simulink library "SunEphemeris_MathWorks"  (R2014b)
settings: Solver=ode45  StartTime=0.0  StopTime=10.0  RelTol=1e-3
undefined symbols (not defined in the file or in its folder): ConfParam
settings Model: Creator=Hp  LastModifiedBy=Hp

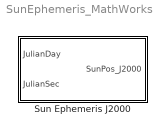
== system SunEphemeris_MathWorks ==
  Sun Ephemeris J2000 : Subsystem

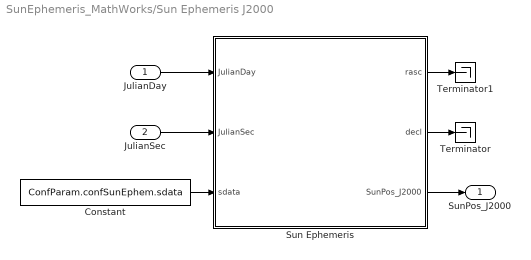
== system SunEphemeris_MathWorks/Sun Ephemeris J2000 ==
  JulianDay : Inport
  JulianSec : Inport  Port=2
  Constant : Constant  Value=ConfParam.confSunEphem.sdata
  Sun Ephemeris : MATLAB Function  TreatAsAtomicUnit=on
  Terminator : Terminator
  Terminator1 : Terminator
  SunPos_J2000 : Outport
  wires:
  Sun Ephemeris/2(decl) -> Terminator/1
  Sun Ephemeris/3(SunPos_J2000) -> SunPos_J2000/1
  JulianDay/1 -> Sun Ephemeris/1(JulianDay)
  Sun Ephemeris/1(rasc) -> Terminator1/1
  Constant/1 -> Sun Ephemeris/3(sdata)
  JulianSec/1 -> Sun Ephemeris/2(JulianSec)

== matlab function SunEphemeris_MathWorks/Sun Ephemeris J2000/Sun Ephemeris ==
  data: JulianDay input; rasc output; JulianSec input; sdata input; decl output; SunPos_J2000 output
function [rasc, decl, SunPos_J2000] = SunEphem (JulianDay, JulianSec, sdata)

% precision ephemeris of the Sun

% input
    
%  jdate = julian ephemeris date

% output

%  rasc = right ascension of the Sun (radians)
%         (0 <= rasc <= 2 pi)
%  decl = declination of the Sun (radians)
%         (-pi/2 <= decl <= pi/2)
%  rsun = eci position vector of the Sun (meters)

% note

%  coordinates are inertial, geocentric,
%  equatorial and true-of-date

% Orbital Mechanics with Matlab

%%%%%%%%%%%%%%%%%%%%%%%%%%%%%%%

sl=zeros(50,1);
sr=zeros(50,1);
sa=zeros(50,1);
sb=zeros(50,1);

% extract data and load arrays

sl(1:1:50) = sdata(1:4:200);
sr(1:1:50) = sdata(2:4:200);
sa(1:1:50) = sdata(3:4:200);
sb(1:1:50) = sdata(4:4:200);

% fundamental time argument
jdate=JulianDay+JulianSec/86400+2.4515445e6;
          
u = (jdate - 2451545) / 3652500;

% compute nutation in longitude

a1 = 2.18 + u * (-3375.7 + u * 0.36);
a2 = 3.51 + u * (125666.39 + u * 0.1);
   
psi = 0.0000001 * (-834 * sin(a1) - 64 * sin(a2));

% compute nutation in obliquity

deps = 0.0000001 * u * (-226938 + u * (-75 + u * (96926 + ...
       u * (-2491 - u * 12104))));

meps = 0.0000001 * (4090928 + 446 * cos(a1) + 28 * cos(a2));
   
eps = meps + deps;
   
seps = sin(eps);
ceps = cos(eps);

dl = 0;
dr = 0;

for i = 1:1:50
    
    w = sa(i) + sb(i) * u;
    
    dl = dl + sl(i) * sin(w);
    
    if (sr(i) ~= 0)
        
       dr = dr + sr(i) * cos(w);
       
    end 
    
end

dl = mod(dl * 0.0000001 + 4.9353929 + 62833.196168 * u, 2.0 * pi);
   
dr = 149597870.691 * (dr * 0.0000001 + 1.0001026);

% geocentric ecliptic position vector of the Sun

rlsun = mod(dl + 0.0000001 * (-993 + 17 * cos(3.1 + 62830.14 * u)) + psi, 2.0 * pi);

rb = 0;

% compute declination and right ascension (radians)

cl = cos(rlsun);
sl = sin(rlsun);
cb = cos(rb);
sb = sin(rb);

decl = asin(ceps * sb + seps * cb * sl);

sra = -seps * sb + ceps * cb * sl;
cra = cb * cl;

rasc = atan3(sra, cra);

SunPos_J2000=zeros(3,1);

% geocentric equatorial position vector of the Sun (kilometers)

SunPos_J2000(1) = dr * cos(rasc) * cos(decl)*1e3;
SunPos_J2000(2) = dr * sin(rasc) * cos(decl)*1e3;
SunPos_J2000(3) = dr * sin(decl)*1e3;

end
